simulink model "PanelwInverter_Backstepping"  (R2016a)
settings: Solver=ode23t  StartTime=0.0  StopTime=30  FixedStep=t_PWM/10  MaxStep=2e-6  RelTol=2e-4
values from neighbouring files (symbols this model uses):
  C1 = t_PWM * (N*Impp)*0.1/ (8 * (N*Vmpp)*0.0001)    [SolarPanelModel.m]
  delta_Il = (N*Impp)*0.1/ 2    [SolarPanelModel.m]
  G = 1000    [SolarPanelModel.m]
  Gr = 1000    [SolarPanelModel.m]
  Isc = G/ Gr * (Iscr + miu_Isc*(Tc - Tr))    (= 9.318625)    [SolarPanelModel.m]
  Iscr = 9.19    [SolarPanelModel.m]
  K = 1.38 * 10^(-23)    (= 1.38e-23)    [SolarPanelModel.m]
  L_inductor = (N*Vo) * t_PWM/ (4 * (N*Impp)*0.01)    [SolarPanelModel.m]
  m = sol(1)    [SolarPanelModel.m]
  miu_Isc = 0.0049    [SolarPanelModel.m]
  miu_Voc = -0.1184    [SolarPanelModel.m]
  N = 3    [SolarPanelModel.m]
  NOCT = 45    [SolarPanelModel.m]
  q = 1.6 * 10^(-19)    (= 1.6e-19)    [SolarPanelModel.m]
  Rs = sol(3)    [SolarPanelModel.m]
  Rsh = sol(2)    [SolarPanelModel.m]
  T = 273.15    [SolarPanelModel.m]
  t_PWM = 20e-6    (= 2e-05)    [SolarPanelModel.m]
  ta = 20    [SolarPanelModel.m]
  Tr = T + 25    (= 298.15)    [SolarPanelModel.m]
  Voc = Vocr + miu_Voc*(Tc - Tr) + m*Vt*log(G/Gr)    [SolarPanelModel.m]
  Vocr = 38.2    [SolarPanelModel.m]
undefined symbols (not defined in the file or in its folder): Cdc_inv, Cp, delta_Ii, g1, GAMA, GREEN, k2, k_A, k_inv, ki_ig, kv_ig, Li, ORANGE, RED, t_int, trigger_signal
libraries: powerlib x33, simulink x6, powerlib_extras x6, powerlib_meascontrol x1
settings Model: Creator=frede  LastModifiedBy=frede
settings DataIOCC: LimitDataPoints=on  SaveFormat=Array
settings HardwareCC: ProdBitPerPointer=32  ProdLargestAtomicFloat=None  ProdIntDivRoundTo=Undefined  ProdEndianess=Unspecified  ProdWordSize=32  ProdHWDeviceType=32-bit Generic
settings ModelReferenceCC: PropagateSignalLabelsOutOfModel=off
settings ConfigComp: CovModelRefEnable=Off

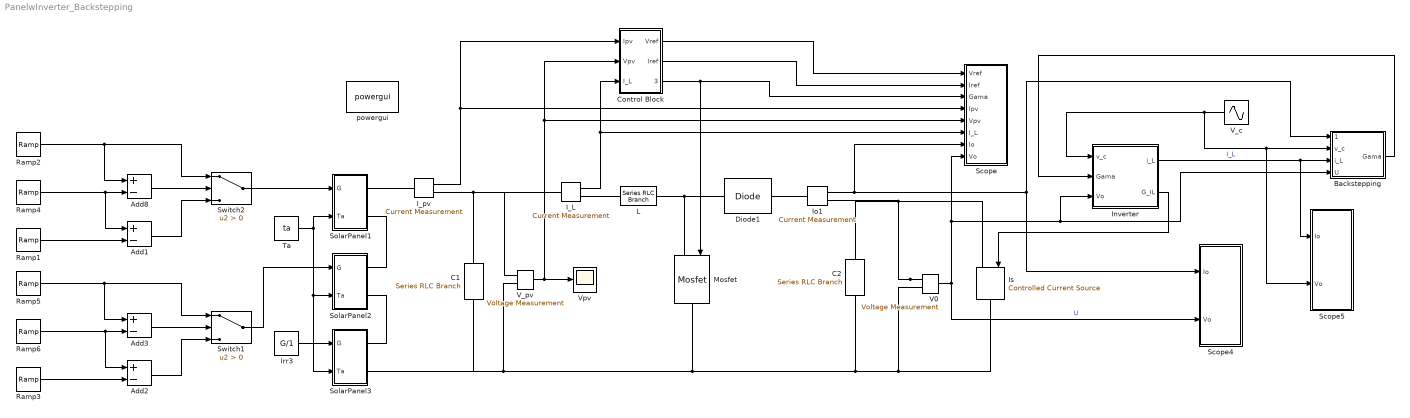
== system PanelwInverter_Backstepping ==
  Add{1..3,8} (4 alike) : Sum  Inputs=+-
  Backstepping : Subsystem
  C1 : powerlib/Elements/Series RLC Branch  LConnTagsString=__new0  RConnTagsString=__new0  BranchType=C  Resistance=Rs  Inductance=1e-3  SetiL0=off  InitialCurrent=0  Capacitance=C1  Setx0=off  InitialVoltage=0  Measurements=None
  C2 : powerlib/Elements/Series RLC Branch  LConnTagsString=__new0  RConnTagsString=__new0  BranchType=C  Resistance=Rs  Inductance=1e-3  SetiL0=off  InitialCurrent=0  Capacitance=Cdc_inv  Setx0=on  InitialVoltage=400  Measurements=None
  Control Block : Subsystem
  Diode1 : powerlib/Power Electronics/Diode  Ron=0.001  Lon=0  Vf=0.001  IC=0  UseSnubber=off  Rs=500  Cs=1e-9  Measurements=off
  I_L : powerlib/Measurements/Current Measurement  PhasorSimulation=off  OutputType=Complex  PSBequivalent=0
  I_pv : powerlib/Measurements/Current Measurement  PhasorSimulation=off  OutputType=Complex  PSBequivalent=0
  Inverter : Subsystem
  Io1 : powerlib/Measurements/Current Measurement  PhasorSimulation=off  OutputType=Complex  PSBequivalent=0
  Irr3 : Constant  Value=G/1
  Is : powerlib/Electrical Sources/Controlled Current Source  Initialize=on  Source_Type=DC  Amplitude=0  Phase=0  Frequency=0  Measurements=None
  L : powerlib/Elements/Series RLC Branch  LConnTagsString=__new0  RConnTagsString=__new0  BranchType=L  Resistance=Rs  Inductance=L_inductor  SetiL0=off  InitialCurrent=0  Capacitance=1e-6  Setx0=off  InitialVoltage=0  Measurements=None
  Mosfet : powerlib/Power Electronics/Mosfet  Ron=0.001  Lon=0  Rd=0.001  Vfd=0  IC=0  Rs=1e3  Cs=1e-9  Measurements=off
  Ramp1 : simulink/Sources/Ramp  slope=31.25  start=t5  X0=0
  Ramp2 : simulink/Sources/Ramp  slope=-31.25  start=t1  X0=g1
  Ramp3 : simulink/Sources/Ramp  slope=25  start=t6  X0=0
  Ramp4 : simulink/Sources/Ramp  slope=31.25  start=-10  X0=0
  Ramp5 : simulink/Sources/Ramp  slope=-25  start=t4  X0=g1
  Ramp6 : simulink/Sources/Ramp  slope=25  start=-20  X0=0
  Scope : Subsystem
  Scope4 : Subsystem
  Scope5 : Subsystem
  SolarPanel1 : Subsystem
  SolarPanel2 : Subsystem
  SolarPanel3 : Subsystem
  Switch1 : Switch  Criteria=u2 > Threshold
  Switch2 : Switch  Criteria=u2 > Threshold
  Ta : Constant  Value=ta
  V0 : powerlib/Measurements/Voltage Measurement  PhasorSimulation=off  OutputType=Complex  PSBequivalent=0
  V_c : Sin  Amplitude=sqrt(2)*230  Frequency=2*pi*50  SampleTime=0
  V_pv : powerlib/Measurements/Voltage Measurement  PhasorSimulation=off  OutputType=Complex  PSBequivalent=0
  Vpv : Scope
  powergui : powerlib/powergui  Priority=1  SimulationMode=Discrete  SolverType=Tustin/Backward Euler (TBE)  SampleTime=t_PWM/10  frequency=60  SPID=off  DisableSnubberDevices=off  DisableRonSwitches=off  DisableVfSwitches=off  SwTol=0  DisplayEquations=off  Interpol=off  ExternalGateDelay=off  methode=off  Ts=10  FunctionMessages=off  echomessages=off  HookPort=off  EnableUseOfTLC=off  x0status=blocks  frequencyindice=0  Pbase=100e6  ErrMax=1e-4  Iterations=50  UnitsV=kV  UnitsW=MW  buscounter=0  RestoreLinks=warning  ResistiveCurrentMeasurement=off  Frange=[0:2:500]  Ylog=off  Xlog=on  ShowGrid=off  save=off  variable=ZData  structure=0  ZoomFFT=off  StartTime=0.0  cycles=1  DisplayStyle=1  fundamental=60  FreqAxis=off  MaxFrequency=1000  frequencyindicesteady=1  RmsSteady=1  display=off
  wires:
  Ta/1 -> SolarPanel1/2(Ta), SolarPanel3/2(Ta), SolarPanel2/2(Ta)
  Irr3/1 -> SolarPanel3/1(G)
  Backstepping/1(Gama) -> Inverter/2(Gama)
  V_c/1 -> Scope5/2(Vo), Backstepping/2(v_c), Inverter/1(v_c)
  V0/1 -> Scope4/2(Vo), Scope/8(Vo), Inverter/3(Vo), Backstepping/4(U)  "U"
  Inverter/1(i_L) -> Backstepping/3(i_L), Scope5/1(Io)  "I_L"
  Inverter/2(G_IL) -> Is/1
  I_L/1 -> Scope/6(I_L), Control Block/3(I_L)
  Control Block/3(Gama) -> Mosfet/1, Scope/3(Gama)
  V_pv/1 -> Vpv/1, Scope/5(Vpv), Control Block/2(Vpv)
  Control Block/1(Vref) -> Scope/1(Vref)
  Control Block/2(Iref) -> Scope/2(Iref)
  Io1/1 -> Scope/7(Io), Scope4/1(Io), Backstepping/1(I_boost)
  I_pv/1 -> Control Block/1(Ipv), Scope/4(Ipv)
  Ramp4/1 -> Add1/1, Add8/2
  Ramp2/1 -> Switch2/1, Add8/1
  Add8/1 -> Switch2/2
  Ramp1/1 -> Add1/2
  Add1/1 -> Switch2/3
  Ramp6/1 -> Add2/1, Add3/2
  Ramp5/1 -> Switch1/1, Add3/1
  Add3/1 -> Switch1/2
  Ramp3/1 -> Add2/2
  Add2/1 -> Switch1/3
  Switch2/1 -> SolarPanel1/1(G)
  Switch1/1 -> SolarPanel2/1(G)
  connections:
  V_pv/LConn1 -- I_L/LConn1 -- C1/LConn1 -- I_pv/RConn1
  V0/LConn2 -- Is/RConn1 -- C2/RConn1 -- Mosfet/RConn1 -- SolarPanel3/RConn2 -- C1/RConn1 -- V_pv/LConn2
  Mosfet/LConn1 -- L/RConn1 -- Diode1/LConn1
  I_L/RConn1 -- L/LConn1
  SolarPanel3/RConn1 -- SolarPanel2/RConn2
  SolarPanel2/RConn1 -- SolarPanel1/RConn2
  SolarPanel1/RConn1 -- I_pv/LConn1
  V0/LConn1 -- Io1/RConn1 -- C2/LConn1 -- Is/LConn1
  Diode1/RConn1 -- Io1/LConn1

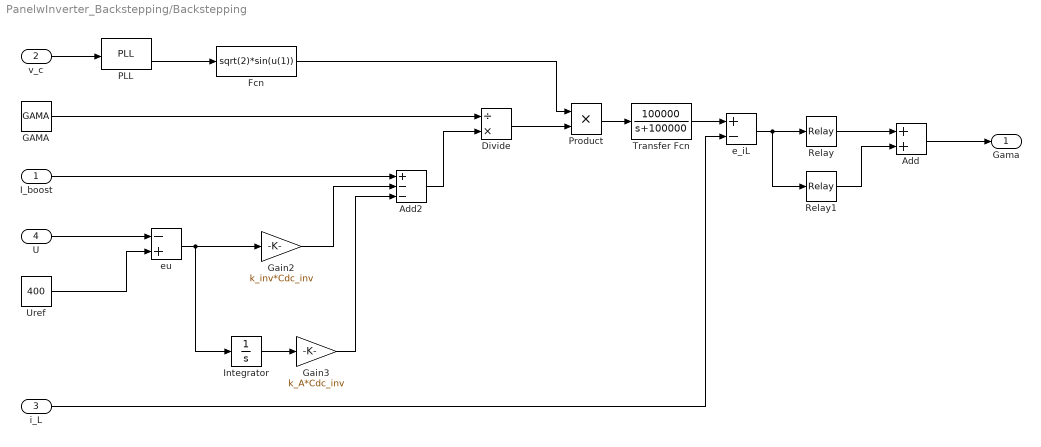
== system PanelwInverter_Backstepping/Backstepping ==
  I_boost : Inport
  v_c : Inport  Port=2
  i_L : Inport  Port=3
  U : Inport  Port=4
  Add : Sum
  Add2 : Sum  Inputs=+--
  Divide : Product  Inputs=/*
  Fcn : Fcn  Expr=sqrt(2)*sin(u(1))
  GAMA : Constant  Value=GAMA
  Gain2 : Gain  Gain=k_inv*Cdc_inv
  Gain3 : Gain  Gain=k_A*Cdc_inv
  Integrator : Integrator  UpperSaturationLimit=30  LowerSaturationLimit=-30
  PLL : powerlib_meascontrol/PLL/PLL  Fmin=45  Par_Init=[0, 50]  ParK=[180, 3200, 1]  TcD=1e-4  MaxRateChangeFreq=12  FilterCutOffFreq=25  Ts=0  AGC=on
  Product : Product
  Relay : Relay  OnSwitchValue=delta_Ii  OffSwitchValue=-delta_Ii  OnOutputValue=0.5  OffOutputValue=-0.5  ZeroCross=off
  Relay1 : Relay  OnSwitchValue=delta_Ii/2  OffSwitchValue=-delta_Ii/2  OnOutputValue=0.5  OffOutputValue=-0.5  ZeroCross=off
  Transfer Fcn : TransferFcn  Numerator=[100000]  Denominator=[1 100000]
  Uref : Constant  Value=400
  e_iL : Sum  Inputs=+-
  eu : Sum  Inputs=-+
  Gama : Outport
  wires:
  e_iL/1 -> Relay1/1, Relay/1
  i_L/1 -> e_iL/2
  Relay/1 -> Add/1
  Relay1/1 -> Add/2
  Add/1 -> Gama/1
  v_c/1 -> PLL/1
  PLL/2 -> Fcn/1
  Product/1 -> Transfer Fcn/1
  Fcn/1 -> Product/1
  eu/1 -> Integrator/1, Gain2/1
  Gain2/1 -> Add2/2
  Add2/1 -> Divide/2
  Uref/1 -> eu/2
  GAMA/1 -> Divide/1
  I_boost/1 -> Add2/1
  Divide/1 -> Product/2
  U/1 -> eu/1
  Integrator/1 -> Gain3/1
  Gain3/1 -> Add2/3
  Transfer Fcn/1 -> e_iL/1

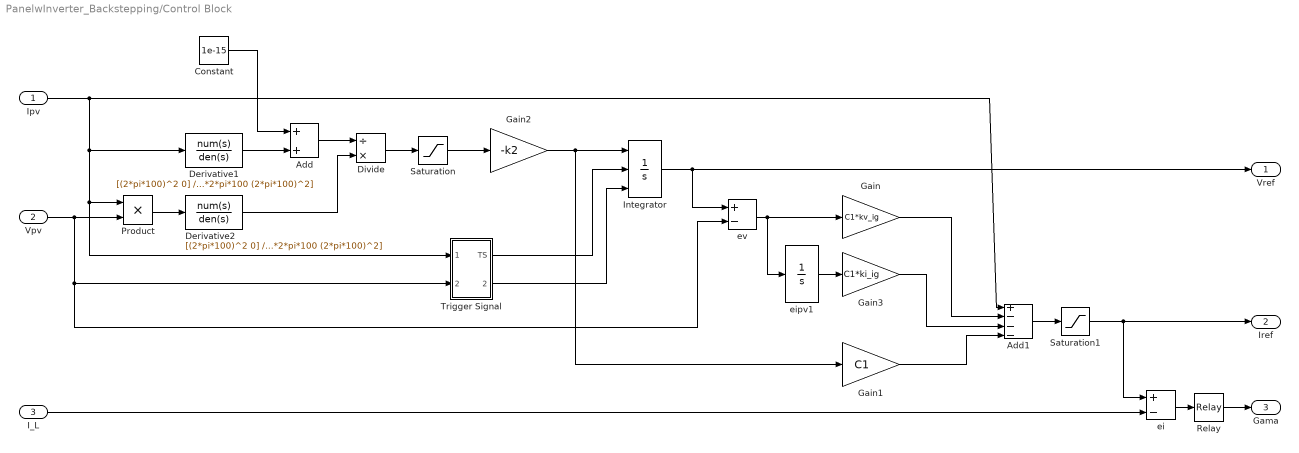
== system PanelwInverter_Backstepping/Control Block ==
  Ipv : Inport
  Vpv : Inport  Port=2
  I_L : Inport  Port=3
  Add : Sum
  Add1 : Sum  Inputs=+---
  Constant : Constant  Value=1e-15
  Derivative1 : TransferFcn  Numerator=[(2*pi*100)^2 0]  Denominator=[1 2*0.7*2*pi*100 (2*pi*100)^2]
  Derivative2 : TransferFcn  Numerator=[(2*pi*100)^2 0]  Denominator=[1 2*0.7*2*pi*100 (2*pi*100)^2]
  Divide : Product  Inputs=/*
  Gain : Gain  Gain=C1*kv_ig
  Gain1 : Gain  Gain=C1
  Gain2 : Gain  Gain=-k2
  Gain3 : Gain  Gain=C1*ki_ig
  Integrator : Integrator  ExternalReset=rising  InitialConditionSource=external  InitialCondition=Voc*0.75  LimitOutput=on  UpperSaturationLimit=Voc*3  LowerSaturationLimit=0
  Product : Product  Inputs=**
  Relay : Relay  OnSwitchValue=delta_Il  OffSwitchValue=-delta_Il
  Saturation : Saturate  UpperLimit=2  LowerLimit=-2
  Saturation1 : Saturate  UpperLimit=Isc*1.2  LowerLimit=0
  Trigger Signal : Subsystem
  ei : Sum  Inputs=+-
  eipv1 : Integrator  UpperSaturationLimit=Voc*N  LowerSaturationLimit=0
  ev : Sum  Inputs=+-
  Vref : Outport
  Iref : Outport  Port=2
  Gama : Outport  Port=3
  wires:
  ev/1 -> eipv1/1, Gain/1
  Gain/1 -> Add1/2
  Gain1/1 -> Add1/4
  Integrator/1 -> ev/1, Vref/1
  eipv1/1 -> Gain3/1
  Gain3/1 -> Add1/3
  Add1/1 -> Saturation1/1
  I_L/1 -> ei/2
  ei/1 -> Relay/1
  Relay/1 -> Gama/1
  Saturation1/1 -> Iref/1, ei/1
  Saturation/1 -> Gain2/1
  Derivative1/1 -> Add/2
  Constant/1 -> Add/1
  Gain2/1 -> Integrator/1, Gain1/1
  Product/1 -> Derivative2/1
  Divide/1 -> Saturation/1
  Add/1 -> Divide/1
  Derivative2/1 -> Divide/2
  Ipv/1 -> Add1/1, Derivative1/1, Trigger Signal/1(Ipv), Product/1
  Vpv/1 -> Trigger Signal/2(Vpv), ev/2, Product/2
  Trigger Signal/1(TS) -> Integrator/2
  Trigger Signal/2(Vref) -> Integrator/3

== system PanelwInverter_Backstepping/Inverter ==
  v_c : Inport
  Gama : Inport  Port=2
  Vo : Inport  Port=3
  Add1 : Sum  Inputs=+-
  Product : Product
  Product1 : Product
  Transfer Fcn : TransferFcn  Denominator=[Li 3]
  i_L : Outport
  G_IL : Outport  Port=2
  wires:
  Add1/1 -> Transfer Fcn/1
  Product/1 -> G_IL/1
  Product1/1 -> Add1/1
  v_c/1 -> Add1/2
  Gama/1 -> Product1/2, Product/1
  Vo/1 -> Product1/1
  Transfer Fcn/1 -> i_L/1, Product/2

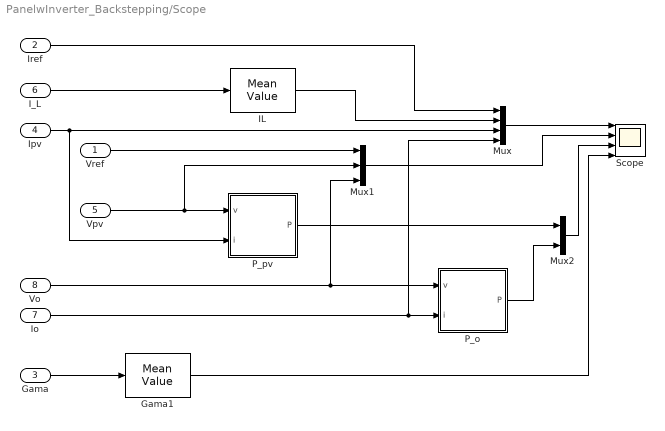
== system PanelwInverter_Backstepping/Scope ==
  Vref : Inport
  Iref : Inport  Port=2
  Gama : Inport  Port=3
  Ipv : Inport  Port=4
  Vpv : Inport  Port=5
  I_L : Inport  Port=6
  Io : Inport  Port=7
  Vo : Inport  Port=8
  Gama1 : powerlib_extras/Measurements/Mean Value  Period=1/1000
  IL : powerlib_extras/Measurements/Mean Value  Period=1/1000
  Mux : Mux
  Mux1 : Mux  Inputs=3
  Mux2 : Mux  Inputs=2
  P_o : Subsystem
  P_pv : Subsystem
  Scope : Scope  NumInputPorts=4
  wires:
  Mux/1 -> Scope/1
  Mux2/1 -> Scope/3
  P_pv/1(P) -> Mux2/1
  Io/1 -> Mux/4, P_o/2(i)
  Mux1/1 -> Scope/2
  Ipv/1 -> Mux/3, P_pv/2(i)
  Vpv/1 -> Mux1/2, P_pv/1(v)
  Vref/1 -> Mux1/1
  P_o/1(P) -> Mux2/2
  I_L/1 -> IL/1
  IL/1 -> Mux/2
  Iref/1 -> Mux/1
  Gama/1 -> Gama1/1
  Gama1/1 -> Scope/4
  Vo/1 -> Mux1/3, P_o/1(v)

== system PanelwInverter_Backstepping/Scope4 ==
  Io : Inport
  Vo : Inport  Port=2
  DC side : Scope  NumInputPorts=3
  P_o : Subsystem
  To Workspace : ToWorkspace  VariableName=Po  SaveFormat=Timeseries  SampleTime=-1
  To Workspace1 : ToWorkspace  VariableName=Vo  SaveFormat=Timeseries  SampleTime=-1
  wires:
  P_o/1(P) -> DC side/3, To Workspace/1
  Io/1 -> DC side/2, P_o/2(i)
  Vo/1 -> To Workspace1/1, DC side/1, P_o/1(v)

== system PanelwInverter_Backstepping/Scope5 ==
  Io : Inport
  Vo : Inport  Port=2
  Grid : Scope  NumInputPorts=3
  P_o : Subsystem
  To Workspace : ToWorkspace  VariableName=Pg  SaveFormat=Timeseries  SampleTime=-1
  To Workspace1 : ToWorkspace  VariableName=Ig  SaveFormat=Timeseries  SampleTime=-1
  wires:
  Io/1 -> To Workspace1/1, Grid/2, P_o/2(i)
  Vo/1 -> Grid/1, P_o/1(v)
  P_o/1(P) -> To Workspace/1, Grid/3

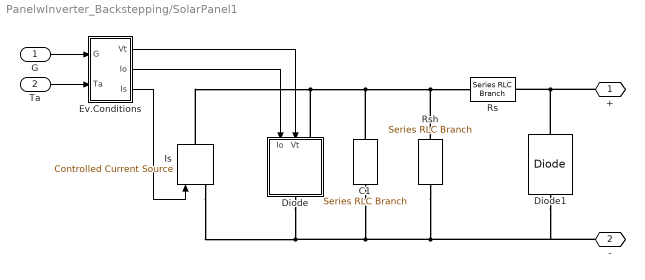
== system PanelwInverter_Backstepping/SolarPanel1 ==
  G : Inport
  Ta : Inport  Port=2
  C1 : powerlib/Elements/Series RLC Branch  LConnTagsString=__new0  RConnTagsString=__new0  BranchType=C  Resistance=Rs  Inductance=1e-3  SetiL0=off  InitialCurrent=0  Capacitance=Cp  Setx0=off  InitialVoltage=0  Measurements=None
  Diode : Subsystem  AncestorBlock=re_lib/Solar/PV Array/Diode Rsh
      mask Display:
      | plot(-75,-50,100,150, [-15 -15 43 -15 -15 -75],[50 8 50 92 50 50], ...
      |     [43 43],[8 94],[100 43], [50 50])
  Diode1 : powerlib/Power Electronics/Diode  Ron=0.001  Lon=0  Vf=0  IC=0  UseSnubber=off  Rs=500  Cs=250e-9  Measurements=off
  Ev.Conditions : Subsystem
  Is : powerlib/Electrical Sources/Controlled Current Source  Initialize=on  Source_Type=DC  Amplitude=0  Phase=0  Frequency=0  Measurements=None
  Rs : powerlib/Elements/Series RLC Branch  LConnTagsString=__new0  RConnTagsString=__new0  BranchType=R  Resistance=Rs  Inductance=1e-3  SetiL0=off  InitialCurrent=0  Capacitance=1e-6  Setx0=off  InitialVoltage=0  Measurements=None
  Rsh : powerlib/Elements/Series RLC Branch  LConnTagsString=__new0  RConnTagsString=__new0  BranchType=R  Resistance=Rsh  Inductance=1e-3  SetiL0=off  InitialCurrent=0  Capacitance=1e-6  Setx0=off  InitialVoltage=0  Measurements=None
  + : PMIOPort  Port=1  Side=Right
  - : PMIOPort  Port=2  Side=Right
  wires:
  G/1 -> Ev.Conditions/1(G)
  Ta/1 -> Ev.Conditions/2(Ta)
  Ev.Conditions/2(Io) -> Diode/1(Io)
  Ev.Conditions/1(Vt) -> Diode/2(Vt)
  Ev.Conditions/3(Is) -> Is/1
  connections:
  Is/RConn1 -- Diode/LConn1 -- C1/LConn1 -- Rsh/LConn1 -- Rs/LConn1
  Rsh/RConn1 -- -/RConn1 -- Diode1/LConn1 -- C1/RConn1 -- Is/LConn1 -- Diode/RConn1
  Diode1/RConn1 -- +/RConn1 -- Rs/RConn1

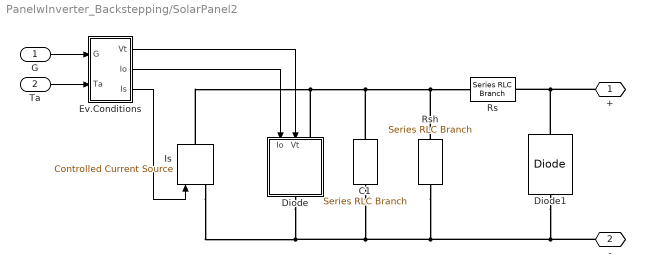
== system PanelwInverter_Backstepping/SolarPanel2 ==
  G : Inport
  Ta : Inport  Port=2
  C1 : powerlib/Elements/Series RLC Branch  LConnTagsString=__new0  RConnTagsString=__new0  BranchType=C  Resistance=Rs  Inductance=1e-3  SetiL0=off  InitialCurrent=0  Capacitance=Cp  Setx0=off  InitialVoltage=0  Measurements=None
  Diode : Subsystem  AncestorBlock=re_lib/Solar/PV Array/Diode Rsh
      mask Display:
      | plot(-75,-50,100,150, [-15 -15 43 -15 -15 -75],[50 8 50 92 50 50], ...
      |     [43 43],[8 94],[100 43], [50 50])
  Diode1 : powerlib/Power Electronics/Diode  Ron=0.001  Lon=0  Vf=0  IC=0  UseSnubber=off  Rs=500  Cs=250e-9  Measurements=off
  Ev.Conditions : Subsystem
  Is : powerlib/Electrical Sources/Controlled Current Source  Initialize=on  Source_Type=DC  Amplitude=0  Phase=0  Frequency=0  Measurements=None
  Rs : powerlib/Elements/Series RLC Branch  LConnTagsString=__new0  RConnTagsString=__new0  BranchType=R  Resistance=Rs  Inductance=1e-3  SetiL0=off  InitialCurrent=0  Capacitance=1e-6  Setx0=off  InitialVoltage=0  Measurements=None
  Rsh : powerlib/Elements/Series RLC Branch  LConnTagsString=__new0  RConnTagsString=__new0  BranchType=R  Resistance=Rsh  Inductance=1e-3  SetiL0=off  InitialCurrent=0  Capacitance=1e-6  Setx0=off  InitialVoltage=0  Measurements=None
  + : PMIOPort  Port=1  Side=Right
  - : PMIOPort  Port=2  Side=Right
  wires:
  G/1 -> Ev.Conditions/1(G)
  Ta/1 -> Ev.Conditions/2(Ta)
  Ev.Conditions/2(Io) -> Diode/1(Io)
  Ev.Conditions/1(Vt) -> Diode/2(Vt)
  Ev.Conditions/3(Is) -> Is/1
  connections:
  Rsh/LConn1 -- Rs/LConn1 -- Is/RConn1 -- Diode/LConn1 -- C1/LConn1
  Is/LConn1 -- Diode/RConn1 -- -/RConn1 -- Diode1/LConn1 -- Rsh/RConn1 -- C1/RConn1
  Diode1/RConn1 -- Rs/RConn1 -- +/RConn1

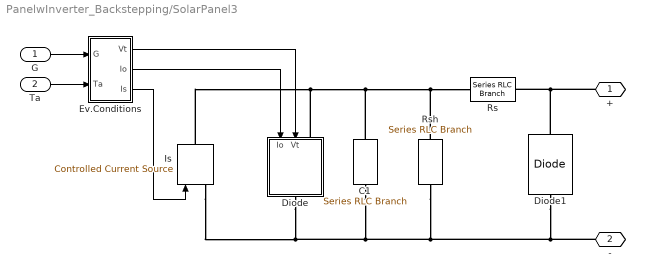
== system PanelwInverter_Backstepping/SolarPanel3 ==
  G : Inport
  Ta : Inport  Port=2
  C1 : powerlib/Elements/Series RLC Branch  LConnTagsString=__new0  RConnTagsString=__new0  BranchType=C  Resistance=Rs  Inductance=1e-3  SetiL0=off  InitialCurrent=0  Capacitance=Cp  Setx0=off  InitialVoltage=0  Measurements=None
  Diode : Subsystem  AncestorBlock=re_lib/Solar/PV Array/Diode Rsh
      mask Display:
      | plot(-75,-50,100,150, [-15 -15 43 -15 -15 -75],[50 8 50 92 50 50], ...
      |     [43 43],[8 94],[100 43], [50 50])
  Diode1 : powerlib/Power Electronics/Diode  Ron=0.001  Lon=0  Vf=0  IC=0  UseSnubber=off  Rs=500  Cs=250e-9  Measurements=off
  Ev.Conditions : Subsystem
  Is : powerlib/Electrical Sources/Controlled Current Source  Initialize=on  Source_Type=DC  Amplitude=0  Phase=0  Frequency=0  Measurements=None
  Rs : powerlib/Elements/Series RLC Branch  LConnTagsString=__new0  RConnTagsString=__new0  BranchType=R  Resistance=Rs  Inductance=1e-3  SetiL0=off  InitialCurrent=0  Capacitance=1e-6  Setx0=off  InitialVoltage=0  Measurements=None
  Rsh : powerlib/Elements/Series RLC Branch  LConnTagsString=__new0  RConnTagsString=__new0  BranchType=R  Resistance=Rsh  Inductance=1e-3  SetiL0=off  InitialCurrent=0  Capacitance=1e-6  Setx0=off  InitialVoltage=0  Measurements=None
  + : PMIOPort  Port=1  Side=Right
  - : PMIOPort  Port=2  Side=Right
  wires:
  G/1 -> Ev.Conditions/1(G)
  Ta/1 -> Ev.Conditions/2(Ta)
  Ev.Conditions/2(Io) -> Diode/1(Io)
  Ev.Conditions/1(Vt) -> Diode/2(Vt)
  Ev.Conditions/3(Is) -> Is/1
  connections:
  Rsh/LConn1 -- Rs/LConn1 -- Is/RConn1 -- Diode/LConn1 -- C1/LConn1
  Is/LConn1 -- Diode/RConn1 -- -/RConn1 -- Diode1/LConn1 -- Rsh/RConn1 -- C1/RConn1
  Diode1/RConn1 -- Rs/RConn1 -- +/RConn1

== system PanelwInverter_Backstepping/Control Block/Trigger Signal ==
  Ipv : Inport
  Vpv : Inport  Port=2
  P_pv : Product
  Scope : Scope
  Scope1 : Scope
  States : Stateflow chart  TreatAsAtomicUnit=on
  TS : Outport
  Vref : Outport  Port=2
  wires:
  Vpv/1 -> P_pv/1, States/1(V_pv)
  Ipv/1 -> P_pv/2
  P_pv/1 -> States/2(P_pv)
  States/1(Light) -> Scope/1
  States/2(Vref) -> Vref/1
  States/3(TS) -> TS/1
  States/4(Pmem) -> Scope1/1

== system PanelwInverter_Backstepping/Scope/P_o ==
  v : Inport
  i : Inport  Port=2
  Mean Value : powerlib_extras/Measurements/Mean Value  Period=1/50
  Product : Product
  P : Outport
  wires:
  Mean Value/1 -> P/1
  Product/1 -> Mean Value/1
  v/1 -> Product/1
  i/1 -> Product/2

== system PanelwInverter_Backstepping/Scope/P_pv ==
  v : Inport
  i : Inport  Port=2
  Mean Value : powerlib_extras/Measurements/Mean Value  Period=1/1000
  Product : Product
  P : Outport
  wires:
  Mean Value/1 -> P/1
  Product/1 -> Mean Value/1
  v/1 -> Product/1
  i/1 -> Product/2

== system PanelwInverter_Backstepping/Scope4/P_o ==
  v : Inport
  i : Inport  Port=2
  Mean Value : powerlib_extras/Measurements/Mean Value  Period=1/50
  Product : Product
  P : Outport
  wires:
  Mean Value/1 -> P/1
  Product/1 -> Mean Value/1
  v/1 -> Product/1
  i/1 -> Product/2

== system PanelwInverter_Backstepping/Scope5/P_o ==
  v : Inport
  i : Inport  Port=2
  Mean Value : powerlib_extras/Measurements/Mean Value  Period=1/50
  Product : Product
  P : Outport
  wires:
  Mean Value/1 -> P/1
  Product/1 -> Mean Value/1
  v/1 -> Product/1
  i/1 -> Product/2

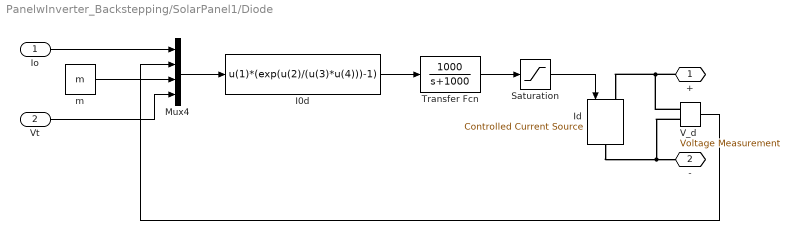
== system PanelwInverter_Backstepping/SolarPanel1/Diode ==
  Io : Inport
  Vt : Inport  Port=2
  I0d : Fcn  Expr=u(1)*(exp(u(2)/(u(3)*u(4)))-1)
  Id : powerlib/Electrical Sources/Controlled Current Source  Initialize=on  Source_Type=DC  Amplitude=0  Phase=0  Frequency=0  Measurements=None
  Mux4 : Mux
  Saturation : Saturate  UpperLimit=Isc  LowerLimit=0
  Transfer Fcn : TransferFcn  Numerator=[1000]  Denominator=[1 1000]
  V_d : powerlib/Measurements/Voltage Measurement  PhasorSimulation=off  OutputType=Complex  PSBequivalent=0
  m : Constant  Value=m
  + : PMIOPort  Port=1  Side=Left
  - : PMIOPort  Port=2  Side=Right
  wires:
  Mux4/1 -> I0d/1
  Io/1 -> Mux4/1
  V_d/1 -> Mux4/2
  m/1 -> Mux4/3
  Vt/1 -> Mux4/4
  I0d/1 -> Transfer Fcn/1
  Transfer Fcn/1 -> Saturation/1
  Saturation/1 -> Id/1
  connections:
  Id/RConn1 -- V_d/LConn2 -- -/RConn1
  +/RConn1 -- V_d/LConn1 -- Id/LConn1

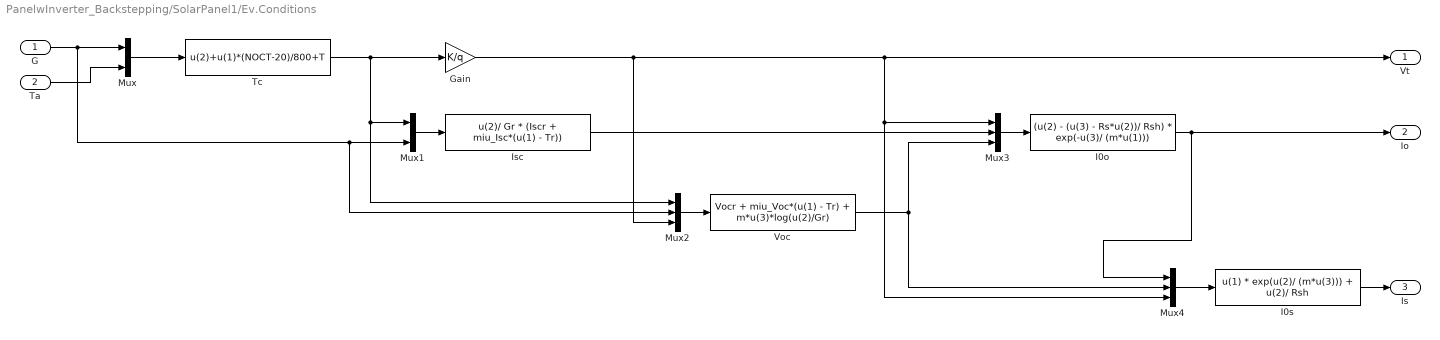
== system PanelwInverter_Backstepping/SolarPanel1/Ev.Conditions ==
  G : Inport
  Ta : Inport  Port=2
  Gain : Gain  Gain=K/q
  I0o : Fcn  Expr=(u(2) - (u(3) - Rs*u(2))/ Rsh) * exp(-u(3)/ (m*u(1)))
  I0s : Fcn  Expr=u(1) * exp(u(2)/ (m*u(3))) + u(2)/ Rsh
  Isc : Fcn  Expr=u(2)/ Gr * (Iscr + miu_Isc*(u(1) - Tr))
  Mux : Mux  Inputs=2
  Mux1 : Mux  Inputs=2
  Mux2 : Mux  Inputs=3
  Mux3 : Mux  Inputs=3
  Mux4 : Mux  Inputs=3
  Tc : Fcn  Expr=u(2)+u(1)*(NOCT-20)/800+T
  Voc : Fcn  Expr=Vocr + miu_Voc*(u(1) - Tr) + m*u(3)*log(u(2)/Gr)
  Vt : Outport
  Io : Outport  Port=2
  Is : Outport  Port=3
  wires:
  Mux1/1 -> Isc/1
  Gain/1 -> Mux2/3, Vt/1, Mux4/3, Mux3/1
  Mux/1 -> Tc/1
  I0s/1 -> Is/1
  Ta/1 -> Mux/2
  G/1 -> Mux/1, Mux2/2, Mux1/2
  Tc/1 -> Mux2/1, Mux1/1, Gain/1
  I0o/1 -> Mux4/1, Io/1
  Mux2/1 -> Voc/1
  Mux3/1 -> I0o/1
  Isc/1 -> Mux3/2
  Voc/1 -> Mux3/3, Mux4/2
  Mux4/1 -> I0s/1

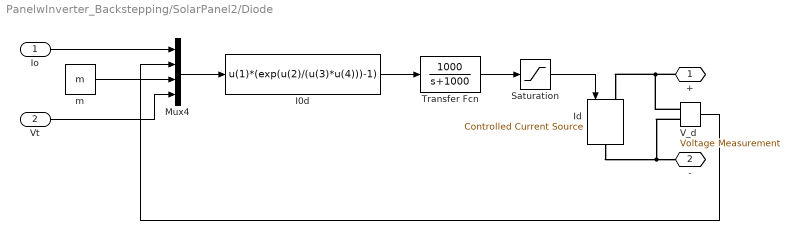
== system PanelwInverter_Backstepping/SolarPanel2/Diode ==
  Io : Inport
  Vt : Inport  Port=2
  I0d : Fcn  Expr=u(1)*(exp(u(2)/(u(3)*u(4)))-1)
  Id : powerlib/Electrical Sources/Controlled Current Source  Initialize=on  Source_Type=DC  Amplitude=0  Phase=0  Frequency=0  Measurements=None
  Mux4 : Mux
  Saturation : Saturate  UpperLimit=Isc  LowerLimit=0
  Transfer Fcn : TransferFcn  Numerator=[1000]  Denominator=[1 1000]
  V_d : powerlib/Measurements/Voltage Measurement  PhasorSimulation=off  OutputType=Complex  PSBequivalent=0
  m : Constant  Value=m
  + : PMIOPort  Port=1  Side=Left
  - : PMIOPort  Port=2  Side=Right
  wires:
  Mux4/1 -> I0d/1
  Io/1 -> Mux4/1
  V_d/1 -> Mux4/2
  m/1 -> Mux4/3
  Vt/1 -> Mux4/4
  I0d/1 -> Transfer Fcn/1
  Transfer Fcn/1 -> Saturation/1
  Saturation/1 -> Id/1
  connections:
  Id/RConn1 -- V_d/LConn2 -- -/RConn1
  +/RConn1 -- V_d/LConn1 -- Id/LConn1

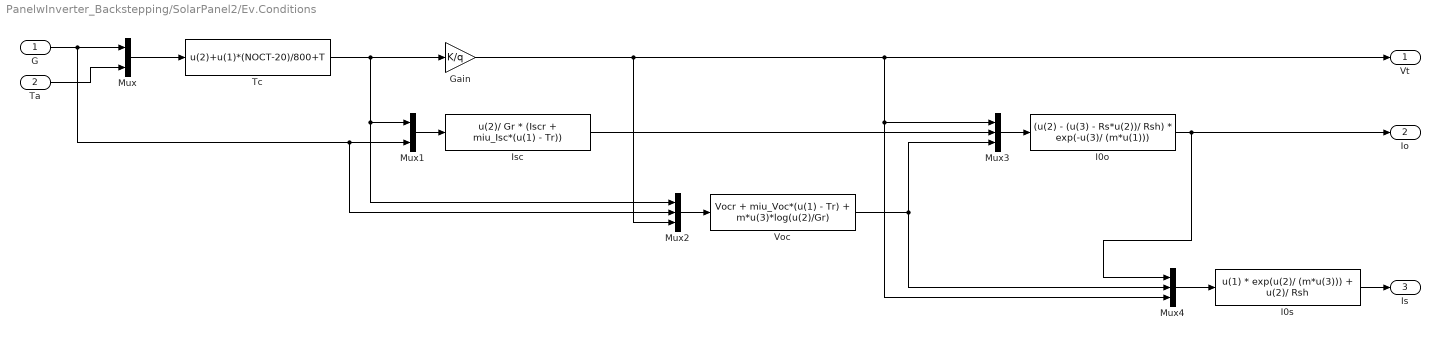
== system PanelwInverter_Backstepping/SolarPanel2/Ev.Conditions ==
  G : Inport
  Ta : Inport  Port=2
  Gain : Gain  Gain=K/q
  I0o : Fcn  Expr=(u(2) - (u(3) - Rs*u(2))/ Rsh) * exp(-u(3)/ (m*u(1)))
  I0s : Fcn  Expr=u(1) * exp(u(2)/ (m*u(3))) + u(2)/ Rsh
  Isc : Fcn  Expr=u(2)/ Gr * (Iscr + miu_Isc*(u(1) - Tr))
  Mux : Mux  Inputs=2
  Mux1 : Mux  Inputs=2
  Mux2 : Mux  Inputs=3
  Mux3 : Mux  Inputs=3
  Mux4 : Mux  Inputs=3
  Tc : Fcn  Expr=u(2)+u(1)*(NOCT-20)/800+T
  Voc : Fcn  Expr=Vocr + miu_Voc*(u(1) - Tr) + m*u(3)*log(u(2)/Gr)
  Vt : Outport
  Io : Outport  Port=2
  Is : Outport  Port=3
  wires:
  Mux1/1 -> Isc/1
  Gain/1 -> Mux2/3, Vt/1, Mux4/3, Mux3/1
  Mux/1 -> Tc/1
  I0s/1 -> Is/1
  Ta/1 -> Mux/2
  G/1 -> Mux/1, Mux2/2, Mux1/2
  Tc/1 -> Mux2/1, Mux1/1, Gain/1
  I0o/1 -> Mux4/1, Io/1
  Mux2/1 -> Voc/1
  Mux3/1 -> I0o/1
  Isc/1 -> Mux3/2
  Voc/1 -> Mux3/3, Mux4/2
  Mux4/1 -> I0s/1

== system PanelwInverter_Backstepping/SolarPanel3/Diode ==
  Io : Inport
  Vt : Inport  Port=2
  I0d : Fcn  Expr=u(1)*(exp(u(2)/(u(3)*u(4)))-1)
  Id : powerlib/Electrical Sources/Controlled Current Source  Initialize=on  Source_Type=DC  Amplitude=0  Phase=0  Frequency=0  Measurements=None
  Mux4 : Mux
  Saturation : Saturate  UpperLimit=Isc  LowerLimit=0
  Transfer Fcn : TransferFcn  Numerator=[1000]  Denominator=[1 1000]
  V_d : powerlib/Measurements/Voltage Measurement  PhasorSimulation=off  OutputType=Complex  PSBequivalent=0
  m : Constant  Value=m
  + : PMIOPort  Port=1  Side=Left
  - : PMIOPort  Port=2  Side=Right
  wires:
  Mux4/1 -> I0d/1
  Io/1 -> Mux4/1
  V_d/1 -> Mux4/2
  m/1 -> Mux4/3
  Vt/1 -> Mux4/4
  I0d/1 -> Transfer Fcn/1
  Transfer Fcn/1 -> Saturation/1
  Saturation/1 -> Id/1
  connections:
  Id/RConn1 -- V_d/LConn2 -- -/RConn1
  +/RConn1 -- V_d/LConn1 -- Id/LConn1

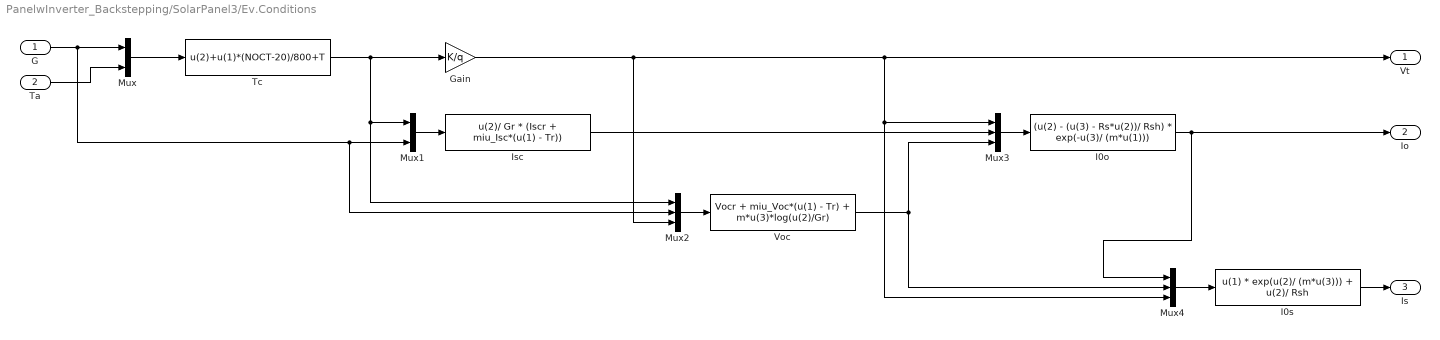
== system PanelwInverter_Backstepping/SolarPanel3/Ev.Conditions ==
  G : Inport
  Ta : Inport  Port=2
  Gain : Gain  Gain=K/q
  I0o : Fcn  Expr=(u(2) - (u(3) - Rs*u(2))/ Rsh) * exp(-u(3)/ (m*u(1)))
  I0s : Fcn  Expr=u(1) * exp(u(2)/ (m*u(3))) + u(2)/ Rsh
  Isc : Fcn  Expr=u(2)/ Gr * (Iscr + miu_Isc*(u(1) - Tr))
  Mux : Mux  Inputs=2
  Mux1 : Mux  Inputs=2
  Mux2 : Mux  Inputs=3
  Mux3 : Mux  Inputs=3
  Mux4 : Mux  Inputs=3
  Tc : Fcn  Expr=u(2)+u(1)*(NOCT-20)/800+T
  Voc : Fcn  Expr=Vocr + miu_Voc*(u(1) - Tr) + m*u(3)*log(u(2)/Gr)
  Vt : Outport
  Io : Outport  Port=2
  Is : Outport  Port=3
  wires:
  Mux1/1 -> Isc/1
  Gain/1 -> Mux2/3, Vt/1, Mux4/3, Mux3/1
  Mux/1 -> Tc/1
  I0s/1 -> Is/1
  Ta/1 -> Mux/2
  G/1 -> Mux/1, Mux2/2, Mux1/2
  Tc/1 -> Mux2/1, Mux1/1, Gain/1
  I0o/1 -> Mux4/1, Io/1
  Mux2/1 -> Voc/1
  Mux3/1 -> I0o/1
  Isc/1 -> Mux3/2
  Voc/1 -> Mux3/3, Mux4/2
  Mux4/1 -> I0s/1

== stateflow chart PanelwInverter_Backstepping/Control Block/Trigger Signal/States ==
  state Setup1
    entry:
    Light = RED;
    Vref = Voc*0.85;
    TS = ON;
  state Setup2
    entry:
    TS = OFF;
  state Setup3
    entry:
    Pmem = P_pv;
    Vmem = V_pv;
    Vref = Voc*0.85*2;
    TS = ON;
  state SteadyState
    entry:
    Light = GREEN;
    delta_P = 0;
    during:
    delta_P = abs(P_pv - Pmem) - Pmem*0.1;
  state NewSearch1
    entry:
    Light = ORANGE;
    Pmem = P_pv;
    Vmem = V_pv;
    if V_pv-Voc < 0
    dir = 1;
    else
    dir = -1;
    end
    Vref = V_pv+dir*Voc*0.85;
    TS = ON;
  state NewSearch2
    entry:
    TS = OFF;
  state NewSearch3
    entry:
    if P_pv > Pmem
    Pmem = P_pv;
    Vmem = V_pv;
    end
    shift = 0;
    if V_pv-Voc < 0
    dir = 1;
    shift = 1;
    end
    Vref = V_pv+dir*Voc*0.85;
    TS = ON;
  state NewSearch3_2
    entry:
    TS = OFF;
  state NewSearch3_1
    entry:
    shift = 0;
  state Setup6
    entry:
    TS = OFF;
  state Setup5
    entry:
    if P_pv > Pmem
    Pmem = P_pv;
    Vmem = V_pv;
    end
    Vref = Voc*0.85*3;
    TS = ON;
  state Setup4
    entry:
    TS = OFF;
    shift = 0;
  state NewSearch5
    entry:
    if P_pv > Pmem
    Pmem = P_pv;
    Vmem = V_pv;
    Vref = Vmem;
    elseif Vmem < 2*Voc && Vmem>Voc
    Vref = 2*Voc*0.85;
    else
    shift = shift + 1;
    Vref = V_pv-dir*Voc*0.85;
    end
    TS = ON;
  state NewSearch4
    entry:
    TS = OFF;
  state NewSearch5_2
    entry:
    TS = OFF;
  state Setup7
    entry:
    if P_pv > Pmem
    Pmem = P_pv;
    Vmem = V_pv;
    Vref = Vmem;
    elseif Vmem > Voc
    Vref = 2*Voc*0.85;
    elseif shift == 0
    shift = shift + 1;
    Vref = Voc*0.85*2;
    else
    shift = shift + 1;
    Vref = Vmem;
    end
    TS = ON;
  state Setup7_2
    entry:
    TS = OFF;
  state NewSearch5_1
    entry:
  state Setup7_1
    entry:
  state NewSearch6
    entry:
    TS = OFF;
  state Setup8
    entry:
    TS = OFF;
    shift = 0;
  state Setup9
    entry:
    Pmem = P_pv;
    Vmem = V_pv;
  (default) -> Setup1
  NewSearch2 -> NewSearch3 : after(t_int,sec)
  NewSearch1 -> NewSearch2 : after(trigger_signal,sec)
  NewSearch3_2 -> NewSearch3 : after(t_int/2,sec)
  SteadyState -> NewSearch1 : [delta_P>0]
  Setup1 -> Setup2 : after(trigger_signal,sec)
  Setup2 -> Setup3 : after(t_int,sec)
  NewSearch3_1 -> NewSearch3_2 : after(trigger_signal,sec)
  Setup9 -> SteadyState
  Setup3 -> Setup4 : after(trigger_signal,sec)
  NewSearch6 -> SteadyState : after(t_int,sec)
  NewSearch3 -> NewSearch3_1 [order 2] : [shift == 1]
  Setup5 -> Setup6 : after(trigger_signal,sec)
  Setup4 -> Setup5 : after(t_int,sec)
  NewSearch3 -> NewSearch4 [order 1] : after(trigger_signal,sec)
  Setup6 -> Setup7 : after(t_int,sec)
  NewSearch4 -> NewSearch5 : after(t_int,sec)
  NewSearch5_2 -> NewSearch5 : after(t_int/2,sec)
  NewSearch5_1 -> NewSearch5_2 : after(trigger_signal,sec)
  Setup7_2 -> Setup7 : after(t_int/2,sec)
  NewSearch5 -> NewSearch5_1 [order 2] : [shift == 1]
  Setup7_1 -> Setup7_2 : after(trigger_signal,sec)
  Setup7 -> Setup7_1 [order 2] : [shift == 1]
  NewSearch5 -> NewSearch6 [order 1] : after(trigger_signal,sec)
  Setup7 -> Setup8 [order 1] : after(trigger_signal,sec)
  Setup8 -> Setup9 : after(t_int,sec)
  data: trigger_signal parameter; Voc parameter; V_pv input; P_pv input; t_int parameter; Light output; Vref output; TS output; Vmem local; RED parameter; ON parameter; OFF parameter; GREEN parameter; delta_P local; ORANGE parameter; dir local; shift local; Pmem output
